simulink model "Controller"  (R2018a)
settings: Solver=ode15s  StartTime=0.0  StopTime=50  MaxStep=0.001  RelTol=1e-3
undefined symbols (not defined in the file or in its folder): d01, d02, I, k1, k2, L0, Lp, q1_0, q1_dot_0, q2_0, q2_dot_0, U1, U2
settings Model: Creator=MJ  LastModifiedBy=MJ

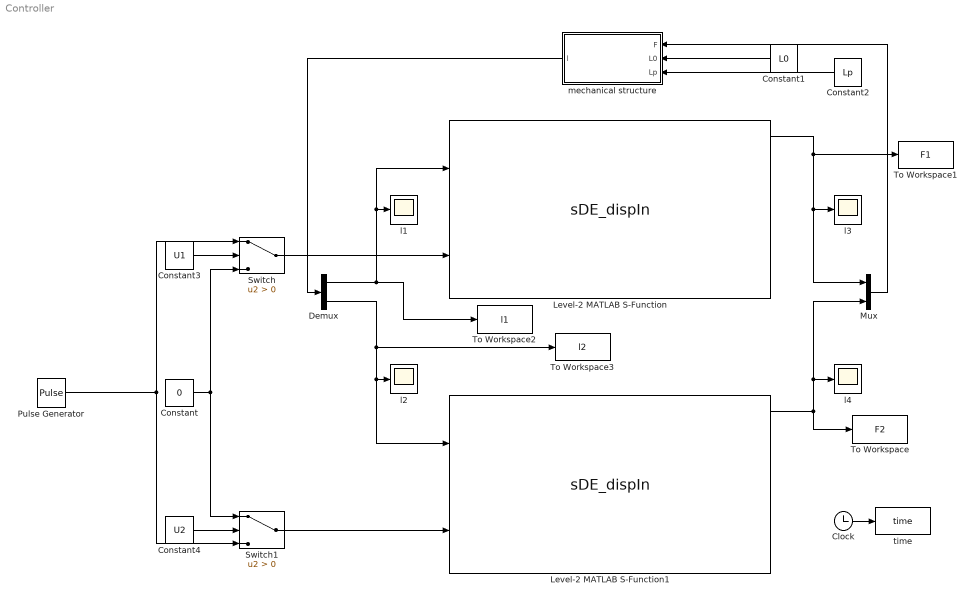
== system Controller ==
  Clock : Clock
  Constant : Constant  Value=0
  Constant1 : Constant  Value=L0
  Constant2 : Constant  Value=Lp
  Constant3 : Constant  Value=U1
  Constant4 : Constant  Value=U2
  Demux : Demux  Outputs=2
  Level-2 MATLAB S-Function : M-S-Function  FunctionName=sDE_dispIn  Parameters=params, initConds
      mask Display:
      | color('black');
      | patch(4*[-1 1 1 -1],1.75*[-1 -1 1 1],[1 1 1]);
      | patch(2*[-1 1 1 -1],1.2*[-1 -1 1 1],[0 0 0]);
      | patch(1.95*[-1 1 1 -1],0.8*[-1 -1 1 1],[1 1 1]);
      | disp('DE Actuator');
      | 
      | color('blue');
      | port_label('input', 1, 'l_1 [m]','texmode','on');
      | port_label('input', 2, 'v [V]','texmode','on');
      | 
      | color('red');
      | port_label('output', 1, 'F_1 [N]','texmode','on');
      | port_label('output', 2, 'x_v [-]','texmode','on');
      | port_label('output', 3, 'q [C]','texmode','on');
      | port_label('output', 4, '\epsilon_1 [-]','texmode','on');
      | port_label('output', 5, '\sigma_1 [Pa]','texmode','on');
      | port_label('output', 6, 'i [A]','texmode','on');
      | port_label('output', 7, 'v_{DE} [V]','texmode','on');
      | port_label('output', 8, 'C [F]','texmode','on');
      | port_label('output', 9, 'E [V/m]','texmode','on');
  Level-2 MATLAB S-Function1 : M-S-Function  FunctionName=sDE_dispIn  Parameters=params, initConds
      mask Display:
      | color('black');
      | patch(4*[-1 1 1 -1],1.75*[-1 -1 1 1],[1 1 1]);
      | patch(2*[-1 1 1 -1],1.2*[-1 -1 1 1],[0 0 0]);
      | patch(1.95*[-1 1 1 -1],0.8*[-1 -1 1 1],[1 1 1]);
      | disp('DE Actuator');
      | 
      | color('blue');
      | port_label('input', 1, 'l_1 [m]','texmode','on');
      | port_label('input', 2, 'v [V]','texmode','on');
      | 
      | color('red');
      | port_label('output', 1, 'F_1 [N]','texmode','on');
      | port_label('output', 2, 'x_v [-]','texmode','on');
      | port_label('output', 3, 'q [C]','texmode','on');
      | port_label('output', 4, '\epsilon_1 [-]','texmode','on');
      | port_label('output', 5, '\sigma_1 [Pa]','texmode','on');
      | port_label('output', 6, 'i [A]','texmode','on');
      | port_label('output', 7, 'v_{DE} [V]','texmode','on');
      | port_label('output', 8, 'C [F]','texmode','on');
      | port_label('output', 9, 'E [V/m]','texmode','on');
  Mux : Mux  Inputs=2
  Pulse Generator : DiscretePulseGenerator  PulseType=Time based  Amplitude=3000  Period=10  PulseWidth=50  PhaseDelay=2.5
  Switch : Switch  Criteria=u2 > Threshold
  Switch1 : Switch  Criteria=u2 > Threshold
  To Workspace : ToWorkspace  VariableName=F2  SampleTime=-1
  To Workspace1 : ToWorkspace  VariableName=F1  SampleTime=-1
  To Workspace2 : ToWorkspace  VariableName=l1  SampleTime=-1
  To Workspace3 : ToWorkspace  VariableName=l2  SampleTime=-1
  l{1..4} (4 alike) : Scope
  mechanical structure : Subsystem
  "time " : ToWorkspace  VariableName=time  SampleTime=-1
  wires:
  mechanical structure/1(l) -> Demux/1
  Mux/1 -> mechanical structure/1(F)
  Demux/1 -> Level-2 MATLAB S-Function/1, l1/1, To Workspace2/1
  Demux/2 -> l2/1, Level-2 MATLAB S-Function1/1, To Workspace3/1
  Level-2 MATLAB S-Function1/1 -> To Workspace/1, l4/1, Mux/2
  Level-2 MATLAB S-Function/1 -> To Workspace1/1, l3/1, Mux/1
  Switch/1 -> Level-2 MATLAB S-Function/2
  Pulse Generator/1 -> Switch1/3, Switch/1
  Constant/1 -> Switch/3, Switch1/1
  Constant1/1 -> mechanical structure/2(L0)
  Constant2/1 -> mechanical structure/3(Lp)
  Clock/1 -> "time "/1
  Switch1/1 -> Level-2 MATLAB S-Function1/2
  Constant3/1 -> Switch/2
  Constant4/1 -> Switch1/2

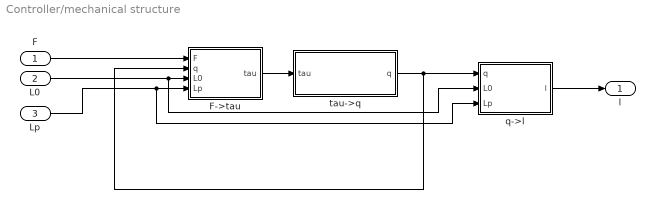
== system Controller/mechanical structure ==
  F : Inport
  L0 : Inport  Port=2
  Lp : Inport  Port=3
  F->tau : MATLAB Function  TreatAsAtomicUnit=on
  q->l : MATLAB Function  TreatAsAtomicUnit=on
  tau->q : Subsystem
  l : Outport
  wires:
  tau->q/1(q) -> q->l/1(q), F->tau/2(q)
  F->tau/1(tau) -> tau->q/1(tau)
  F/1 -> F->tau/1(F)
  q->l/1(l) -> l/1
  L0/1 -> q->l/2(L0), F->tau/3(L0)
  Lp/1 -> q->l/3(Lp), F->tau/4(Lp)

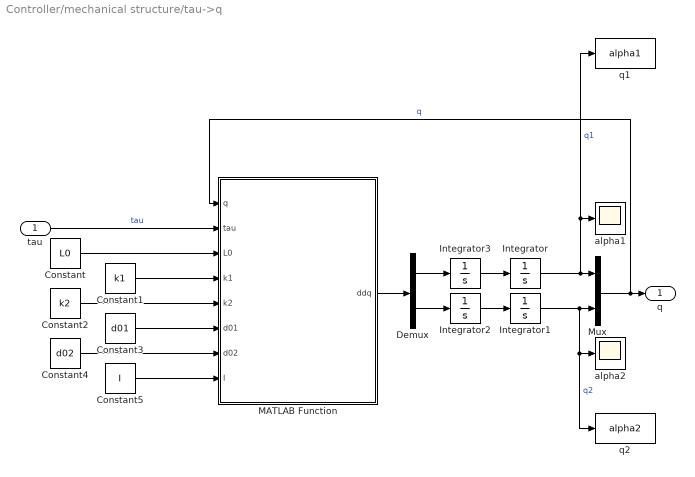
== system Controller/mechanical structure/tau->q ==
  tau : Inport
  Constant : Constant  Value=L0
  Constant1 : Constant  Value=k1
  Constant2 : Constant  Value=k2
  Constant3 : Constant  Value=d01
  Constant4 : Constant  Value=d02
  Constant5 : Constant  Value=I
  Demux : Demux  Outputs=2
  Integrator : Integrator  InitialCondition=q1_0
  Integrator1 : Integrator  InitialCondition=q2_0
  Integrator2 : Integrator  InitialCondition=q2_dot_0
  Integrator3 : Integrator  InitialCondition=q1_dot_0
  MATLAB Function : MATLAB Function  TreatAsAtomicUnit=on
  Mux : Mux  Inputs=2
  alpha1 : Scope
  alpha2 : Scope
  q1 : ToWorkspace  VariableName=alpha1  SampleTime=-1
  q2 : ToWorkspace  VariableName=alpha2  SampleTime=-1
  q : Outport
  wires:
  Integrator3/1 -> Integrator/1
  tau/1 -> MATLAB Function/2(tau)  "tau"
  Integrator2/1 -> Integrator1/1
  Integrator/1 -> q1/1, alpha1/1, Mux/1  "q1"
  Integrator1/1 -> q2/1, alpha2/1, Mux/2  "q2"
  Mux/1 -> MATLAB Function/1(q), q/1  "q"
  MATLAB Function/1(ddq) -> Demux/1
  Demux/1 -> Integrator3/1
  Demux/2 -> Integrator2/1
  Constant/1 -> MATLAB Function/3(L0)
  Constant1/1 -> MATLAB Function/4(k1)
  Constant2/1 -> MATLAB Function/5(k2)
  Constant3/1 -> MATLAB Function/6(d01)
  Constant4/1 -> MATLAB Function/7(d02)
  Constant5/1 -> MATLAB Function/8(I)

== matlab function Controller/mechanical structure/q->l ==
  data: q input size=2; l output size=2; L0 input; Lp input
function l = fcn(q,L0,Lp)

q1 = q(1);
q2 = q(2);

l = [(((2^(1/2)*L0)/2 - L0*cos(q1))^2 + (Lp + (2^(1/2)*L0)/2 - L0*sin(q1))^2)^(1/2);
 (((2^(1/2)*L0)/2 - L0*cos(q2))^2 + (Lp + (2^(1/2)*L0)/2 - L0*sin(q2))^2)^(1/2)];

== matlab function Controller/mechanical structure/F->tau ==
  data: F input; tau output; q input; L0 input; Lp input
function tau = fcn(F,q,L0,Lp)


q1 = q(1);
q2 = q(2);



J = [
    [ -(L0*(2*Lp*cos(q1) + 2^(1/2)*L0*cos(q1) - 2^(1/2)*L0*sin(q1)))/((2*Lp + 2^(1/2)*L0 - 2*L0*sin(q1))^2 + L0^2*(2*cos(q1) - 2^(1/2))^2)^(1/2),                                                                                                                                          0];
    [                                                                                                                                          0, -(L0*(2*Lp*cos(q2) + 2^(1/2)*L0*cos(q2) - 2^(1/2)*L0*sin(q2)))/((2*Lp + 2^(1/2)*L0 - 2*L0*sin(q2))^2 + L0^2*(2*cos(q2) - 2^(1/2))^2)^(1/2)]
    ];

tau = -J'*F;

== matlab function Controller/mechanical structure/tau->q/MATLAB Function ==
  data: q input size=2; ddq output size=2; tau input size=2; L0 input; k1 input; k2 input; d01 input; d02 input; I input
function ddq = fcn(q,tau,L0,k1,k2,d01,d02,I)

q1 = q(1);
q2 = q(2);

tau1 = tau(1);
tau2 = tau(2);

ddq1 = (tau1+(2^(1/2)*L0^2*k1*sin(q1 + q2)*(2*d01 - 2^(1/2)*(-L0^2*(cos(q1 + q2) - 1))^(1/2)))/(8*(-L0^2*(cos(q1 + q2) - 1))^(1/2)) - (2^(1/2)*L0^2*k2*(d02 - 2^(1/2)*(L0^2*(2*sin(pi/9) + cos(q1 + q2 + (2*pi)/9) - 2*sin(q1 + q2 + pi/9) - cos(q1 + q2) + 2))^(1/2))*(2*cos(q1 + q2 + pi/9) + sin(q1 + q2 + (2*pi)/9) - sin(q1 + q2)))/(2*(L0^2*(2*sin(pi/9) + cos(q1 + q2 + (2*pi)/9) - 2*sin(q1 + q2 + pi/9) - cos(q1 + q2) + 2))^(1/2)))/I;
ddq2 = (tau2+(2^(1/2)*L0^2*k1*sin(q1 + q2)*(2*d01 - 2^(1/2)*(-L0^2*(cos(q1 + q2) - 1))^(1/2)))/(8*(-L0^2*(cos(q1 + q2) - 1))^(1/2)) - (2^(1/2)*L0^2*k2*(d02 - 2^(1/2)*(L0^2*(2*sin(pi/9) + cos(q1 + q2 + (2*pi)/9) - 2*sin(q1 + q2 + pi/9) - cos(q1 + q2) + 2))^(1/2))*(2*cos(q1 + q2 + pi/9) + sin(q1 + q2 + (2*pi)/9) - sin(q1 + q2)))/(2*(L0^2*(2*sin(pi/9) + cos(q1 + q2 + (2*pi)/9) - 2*sin(q1 + q2 + pi/9) - cos(q1 + q2) + 2))^(1/2)))/I;

ddq = [ddq1;ddq2];
